simulink model "three_ph_control_power_motor"  (R2016b)
settings: Solver=VariableStepAuto  StartTime=0.0  StopTime=1  RelTol=1e-3
libraries: powerlib x9
settings Model: Creator=Yash Bansod  LastModifiedBy=Yash Bansod

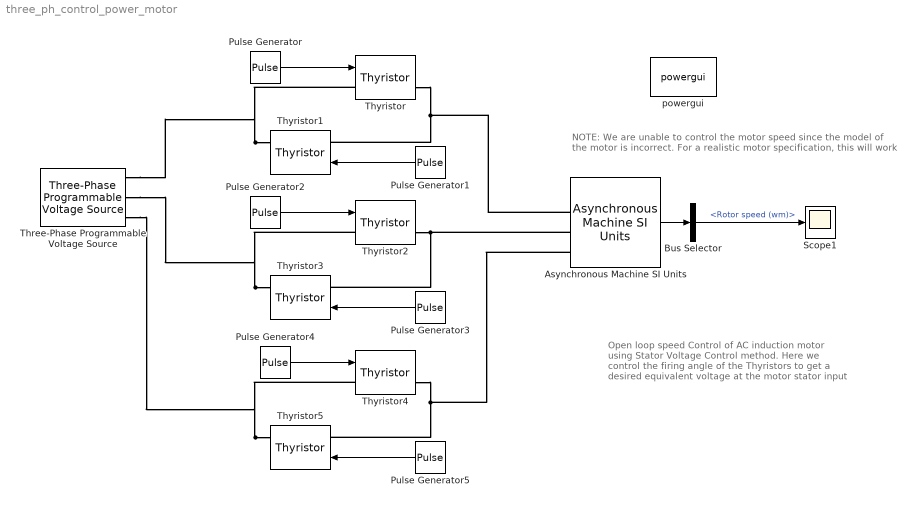
== system three_ph_control_power_motor ==
  note: NOTE:
      | We are unable to control the motor speed since the model of the
      | motor is incorrect. For a realistic motor specification, this will work
  note: Open loop speed Control of AC induction motor
      | using Stator Voltage Control method.
      | Here we control the firing angle of the Thyristors
      | to get a desired equivalent voltage at the motor
      | stator input
  Asynchronous Machine SI Units : powerlib/Machines/Asynchronous Machine SI Units  RotorType=Squirrel-cage  PresetModel=No  MechanicalLoad=Torque Tm  ShowDetailedParameters=on  ReferenceFrame=Rotor  Units=SI  MeasurementBus=off  NominalParameters=[1.845e+04 400 50]  Stator=[0.5968 0.0003495]  Rotor=[0.6258 0.0005473]  Cage1=[0.4155 0.002066]  Cage2=[0.4168 0.0003495]  Lm=0.0354  Mechanical=[0.05 0.005879 2]  PolePairs=2  InitialConditions=[0 0 0 0 0 0 0 0]  SimulateSaturation=off  Saturation=[14.03593122, 27.81365428, 53.79336849, 72.68890987, 97.98006896, 148.6815601, 215.7428561, 302.9841135, 428.7778367 ; 230, 322, 414, 460, 506, 552, 598, 644, 690]  LoadFlowParameters=1492000  TsPowergui=0  TsBlock=-1  IterativeModel=Trapezoidal non iterative  IterativeDiscreteModel=Trapezoidal non iterative  Pmec=1.492e+006
  Bus Selector : BusSelector  OutputSignals=Mechanical.Rotor speed (wm)
  Pulse Generator : DiscretePulseGenerator  PulseType=Time based  Amplitude=10  Period=0.02  PulseWidth=5  PhaseDelay=0+(0.02/9)
  Pulse Generator1 : DiscretePulseGenerator  PulseType=Time based  Amplitude=10  Period=0.02  PulseWidth=5  PhaseDelay=0.01+(0.02/9)
  Pulse Generator2 : DiscretePulseGenerator  PulseType=Time based  Amplitude=10  Period=0.02  PulseWidth=5  PhaseDelay=(0.02/3)+(0.02/9)
  Pulse Generator3 : DiscretePulseGenerator  PulseType=Time based  Amplitude=10  Period=0.02  PulseWidth=5  PhaseDelay=0.01+(0.02/3)+(0.02/9)
  Pulse Generator4 : DiscretePulseGenerator  PulseType=Time based  Amplitude=10  Period=0.02  PulseWidth=5  PhaseDelay=(0.04/3)+(0.02/9)
  Pulse Generator5 : DiscretePulseGenerator  PulseType=Time based  Amplitude=10  Period=0.02  PulseWidth=5  PhaseDelay=0.01+(0.04/3)+(0.02/9)
  Scope1 : Scope
  Three-Phase Programmable Voltage Source : powerlib/Electrical Sources/Three-Phase Programmable Voltage Source  PositiveSequence="[490  0 50]"  VariationEntity=None  VariationType=Table of time-amplitude pairs  VariationTypeAlt=Step  VariationStep=0.5  VariationRate=10  VariationMagnitude=0.3  VariationFrequency=2  VariationTiming=[1 2]  VariationPhaseA=off  Amplitudes=[1 0.8 1.2 1.0]  TimeValues=[0 0.1 0.15 0.2]  HarmonicGeneration=off  HarmonicA=[3 0.2 -25 0]  HarmonicB=[2 0.15 35 2]  Timing="[0.05  3]"  BusType=swing  Pref=0  Qref=0  Qmin=-inf  Qmax=inf
  Thyristor{,1..5} (6 alike) : powerlib/Power Electronics/Thyristor  Ron=0.001  Lon=0  Vf=0.8  IC=0  Rs=500  Cs=250e-9  Measurements=on
  powergui : powerlib/powergui  Priority=1  SimulationMode=Continuous  SolverType=Tustin/Backward Euler (TBE)  SampleTime=50e-6  frequency=60  SPID=off  DisableSnubberDevices=off  DisableRonSwitches=off  DisableVfSwitches=off  SwTol=0  DisplayEquations=off  Interpol=off  ExternalGateDelay=off  methode=off  Ts=10  FunctionMessages=off  echomessages=off  HookPort=off  EnableUseOfTLC=off  x0status=blocks  frequencyindice=50  Pbase=100e6  ErrMax=1e-4  Iterations=50  UnitsV=kV  UnitsW=MW  buscounter=0  RestoreLinks=warning  ResistiveCurrentMeasurement=off  Frange=[0:2:500]  Ylog=off  Xlog=on  ShowGrid=off  save=off  variable=ZData  structure=0  ZoomFFT=off  StartTime=0.0  cycles=1  DisplayStyle=1  fundamental=60  FreqAxis=off  MaxFrequency=1000  frequencyindicesteady=1  RmsSteady=1  display=off
  wires:
  Bus Selector/1 -> Scope1/1  "<Rotor speed (wm)>"
  Asynchronous Machine SI Units/1 -> Bus Selector/1
  Pulse Generator/1 -> Thyristor/1
  Pulse Generator1/1 -> Thyristor1/1
  Pulse Generator3/1 -> Thyristor3/1
  Pulse Generator5/1 -> Thyristor5/1
  Pulse Generator4/1 -> Thyristor4/1
  Pulse Generator2/1 -> Thyristor2/1
  connections:
  Thyristor1/RConn1 -- Three-Phase Programmable Voltage Source/RConn1 -- Thyristor/LConn1
  Thyristor/RConn1 -- Asynchronous Machine SI Units/LConn1 -- Thyristor1/LConn1
  Thyristor3/RConn1 -- Three-Phase Programmable Voltage Source/RConn2 -- Thyristor2/LConn1
  Thyristor2/RConn1 -- Thyristor3/LConn1 -- Asynchronous Machine SI Units/LConn2
  Thyristor5/RConn1 -- Three-Phase Programmable Voltage Source/RConn3 -- Thyristor4/LConn1
  Thyristor4/RConn1 -- Asynchronous Machine SI Units/LConn3 -- Thyristor5/LConn1
